simulink model "monitor1"  (R2018a)
settings: Solver=VariableStepAuto  StartTime=0.0  StopTime=10.0  RelTol=1e-3
values from neighbouring files (symbols this model uses):
  data = curs.Data    [datetime_query.m]    (also in datetime_query1.m; db1.m; db2.m)
undefined symbols (not defined in the file or in its folder): height
libraries: sldrtlib x1
settings Model: Creator=sukri  LastModifiedBy=sukri
settings DataIOCC: ExternalInput=ds  LoadExternalInput=on  ReturnWorkspaceOutputs=on

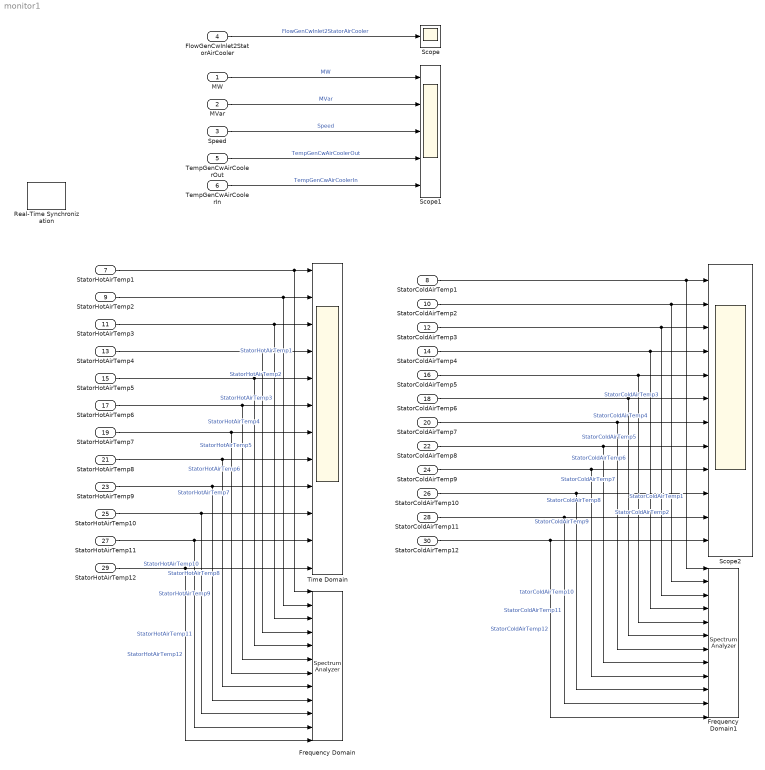
== system monitor1 ==
  MW : Inport  SampleTime=1/(0.1*height(data))
  MVar : Inport  Port=2  SampleTime=1/(0.1*height(data))
  Speed : Inport  Port=3  SampleTime=1/(0.1*height(data))
  FlowGenCwInlet2StatorAirCooler : Inport  Port=4  SampleTime=1/(0.1*height(data))
  TempGenCwAirCoolerOut : Inport  Port=5  SampleTime=1/(0.1*height(data))
  TempGenCwAirCoolerIn : Inport  Port=6  SampleTime=1/(0.1*height(data))
  StatorHotAirTemp1 : Inport  Port=7  SampleTime=1/(0.1*height(data))
  StatorColdAirTemp1 : Inport  Port=8  SampleTime=1/(0.1*height(data))
  StatorHotAirTemp2 : Inport  Port=9  SampleTime=1/(0.1*height(data))
  StatorColdAirTemp2 : Inport  Port=10  SampleTime=1/(0.1*height(data))
  StatorHotAirTemp3 : Inport  Port=11  SampleTime=1/(0.1*height(data))
  StatorColdAirTemp3 : Inport  Port=12  SampleTime=1/(0.1*height(data))
  StatorHotAirTemp4 : Inport  Port=13  SampleTime=1/(0.1*height(data))
  StatorColdAirTemp4 : Inport  Port=14  SampleTime=1/(0.1*height(data))
  StatorHotAirTemp5 : Inport  Port=15  SampleTime=1/(0.1*height(data))
  StatorColdAirTemp5 : Inport  Port=16  SampleTime=1/(0.1*height(data))
  StatorHotAirTemp6 : Inport  Port=17  SampleTime=1/(0.1*height(data))
  StatorColdAirTemp6 : Inport  Port=18  SampleTime=1/(0.1*height(data))
  StatorHotAirTemp7 : Inport  Port=19  SampleTime=1/(0.1*height(data))
  StatorColdAirTemp7 : Inport  Port=20  SampleTime=1/(0.1*height(data))
  StatorHotAirTemp8 : Inport  Port=21  SampleTime=1/(0.1*height(data))
  StatorColdAirTemp8 : Inport  Port=22  SampleTime=1/(0.1*height(data))
  StatorHotAirTemp9 : Inport  Port=23  SampleTime=1/(0.1*height(data))
  StatorColdAirTemp9 : Inport  Port=24  SampleTime=1/(0.1*height(data))
  StatorHotAirTemp10 : Inport  Port=25  SampleTime=1/(0.1*height(data))
  StatorColdAirTemp10 : Inport  Port=26  SampleTime=1/(0.1*height(data))
  StatorHotAirTemp11 : Inport  Port=27  SampleTime=1/(0.1*height(data))
  StatorColdAirTemp11 : Inport  Port=28  SampleTime=1/(0.1*height(data))
  StatorHotAirTemp12 : Inport  Port=29  SampleTime=1/(0.1*height(data))
  StatorColdAirTemp12 : Inport  Port=30  SampleTime=1/(0.1*height(data))
  Frequency Domain : SpectrumAnalyzer  NumInputPorts=12
  Frequency Domain1 : SpectrumAnalyzer  NumInputPorts=12
  Real-Time Synchronization : sldrtlib/Real-Time Synchronization  SampleTime=1  MaxMissedTicks=10  ShowMissedTicks=off  YieldWhenWaiting=off
  Scope : Scope
  Scope1 : Scope  NumInputPorts=5
  Scope2 : Scope  NumInputPorts=12
  Time Domain : Scope  NumInputPorts=12
  wires:
  MW/1 -> Scope1/1  "MW"
  MVar/1 -> Scope1/2  "MVar"
  Speed/1 -> Scope1/3  "Speed"
  FlowGenCwInlet2StatorAirCooler/1 -> Scope/1  "FlowGenCwInlet2StatorAirCooler"
  TempGenCwAirCoolerOut/1 -> Scope1/4  "TempGenCwAirCoolerOut"
  TempGenCwAirCoolerIn/1 -> Scope1/5  "TempGenCwAirCoolerIn"
  StatorHotAirTemp1/1 -> Frequency Domain/1, Time Domain/1  "StatorHotAirTemp1"
  StatorHotAirTemp2/1 -> Frequency Domain/2, Time Domain/2  "StatorHotAirTemp2"
  StatorHotAirTemp3/1 -> Frequency Domain/3, Time Domain/3  "StatorHotAirTemp3"
  StatorHotAirTemp4/1 -> Frequency Domain/4, Time Domain/4  "StatorHotAirTemp4"
  StatorHotAirTemp5/1 -> Frequency Domain/5, Time Domain/5  "StatorHotAirTemp5"
  StatorHotAirTemp6/1 -> Frequency Domain/6, Time Domain/6  "StatorHotAirTemp6"
  StatorHotAirTemp7/1 -> Frequency Domain/7, Time Domain/7  "StatorHotAirTemp7"
  StatorHotAirTemp8/1 -> Frequency Domain/8, Time Domain/8  "StatorHotAirTemp8"
  StatorHotAirTemp9/1 -> Frequency Domain/9, Time Domain/9  "StatorHotAirTemp9"
  StatorHotAirTemp10/1 -> Frequency Domain/10, Time Domain/10  "StatorHotAirTemp10"
  StatorHotAirTemp11/1 -> Frequency Domain/11, Time Domain/11  "StatorHotAirTemp11"
  StatorHotAirTemp12/1 -> Frequency Domain/12, Time Domain/12  "StatorHotAirTemp12"
  StatorColdAirTemp12/1 -> Frequency Domain1/12, Scope2/12  "StatorColdAirTemp12"
  StatorColdAirTemp11/1 -> Frequency Domain1/11, Scope2/11  "StatorColdAirTemp11"
  StatorColdAirTemp1/1 -> Frequency Domain1/1, Scope2/1  "StatorColdAirTemp1"
  StatorColdAirTemp2/1 -> Frequency Domain1/2, Scope2/2  "StatorColdAirTemp2"
  StatorColdAirTemp3/1 -> Frequency Domain1/3, Scope2/3  "StatorColdAirTemp3"
  StatorColdAirTemp4/1 -> Frequency Domain1/4, Scope2/4  "StatorColdAirTemp4"
  StatorColdAirTemp5/1 -> Frequency Domain1/5, Scope2/5  "StatorColdAirTemp5"
  StatorColdAirTemp6/1 -> Frequency Domain1/6, Scope2/6  "StatorColdAirTemp6"
  StatorColdAirTemp7/1 -> Frequency Domain1/7, Scope2/7  "StatorColdAirTemp7"
  StatorColdAirTemp8/1 -> Frequency Domain1/8, Scope2/8  "StatorColdAirTemp8"
  StatorColdAirTemp9/1 -> Frequency Domain1/9, Scope2/9  "StatorColdAirTemp9"
  StatorColdAirTemp10/1 -> Frequency Domain1/10, Scope2/10  "tatorColdAirTemp10"
